simulink model "model"  (Simulink 7.5)
settings: Solver=ode23t  StartTime=0.0  StopTime=1  RelTol=1e-3
InitFcn:
  | sfunction_build
values from neighbouring files (symbols this model uses):
  D = 0.0001    [parameters.m]
  fx = 76.4e-3    (= 0.0764)    [parameters.m]
  J = 0.0001    [parameters.m]
  Lm = 0.0125    [parameters.m]
  P = 8    [parameters.m]
  Rs = 6.4    [parameters.m]
settings Model: Creator=mfilippa  LastModifiedBy=User
settings DebuggingCC: AlgebraicLoopMsg=error

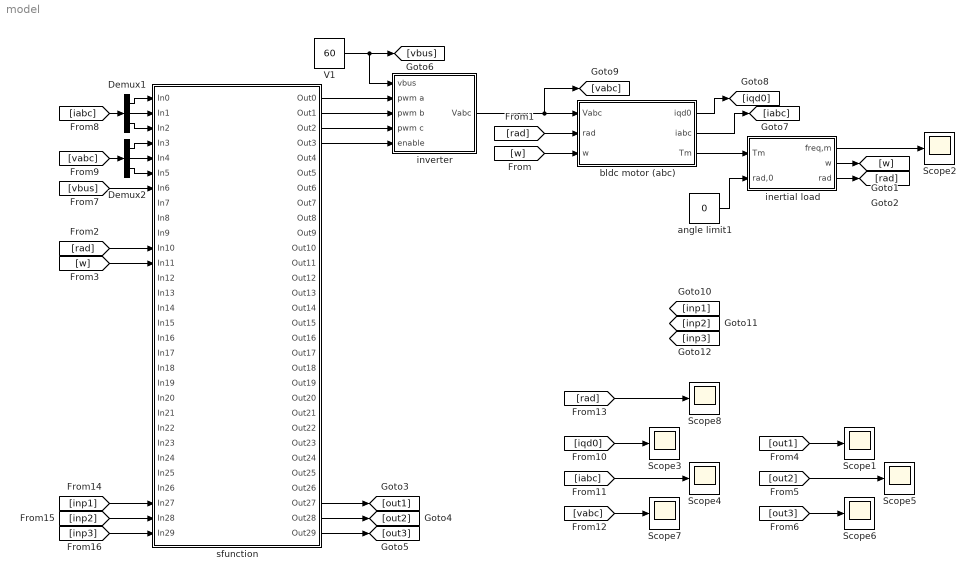
== system model ==
  Demux1 : Demux  Outputs=3
  Demux2 : Demux  Outputs=3
  Scope{1..8} (8 alike) : Scope
      Scope1 settings: YMin=8090  YMax=8230
      Scope3 settings: TimeRange=0.1722129783693844  YMin=-0.0402777777777777  YMax=0.06064814814814822  SaveName=ScopeData2
      Scope4 settings: SaveName=ScopeData3
      Scope5 settings: TimeRange=1.390547243523832e-005  YMin=7709.094650205756  YMax=7968.73799725651  SaveName=ScopeData4
      Scope6 settings: SaveName=ScopeData5
      Scope7 settings: SaveName=ScopeData6
      Scope8 settings: SaveName=ScopeData7
  V1 : Constant  Value=60
  angle limit1 : Constant  Value=0
  bldc motor (abc) : Subsystem
  inertial load : Subsystem
  inverter : Subsystem
  sfunction : Subsystem
  wires:
  V1/1 -> inverter/1(vbus), [vbus]
  sfunction/1(Out0) -> inverter/2(pwm a)
  sfunction/2(Out1) -> inverter/3(pwm b)
  sfunction/3(Out2) -> inverter/4(pwm c)
  sfunction/4(Out3) -> inverter/5(enable)
  [out1] -> Scope1/1
  inverter/1(Vabc) -> bldc motor (abc)/1(Vabc), [vabc]
  bldc motor (abc)/3(Tm) -> inertial load/1(Tm)
  [w] -> bldc motor (abc)/3(w)
  [rad] -> bldc motor (abc)/2(rad)
  inertial load/2(w) -> [w]
  inertial load/3(rad) -> [rad]
  [rad] -> sfunction/11(In10)
  [w] -> sfunction/12(In11)
  sfunction/30(Out29) -> [out3]
  sfunction/29(Out28) -> [out2]
  sfunction/28(Out27) -> [out1]
  [out2] -> Scope5/1
  [out3] -> Scope6/1
  [vbus] -> sfunction/7(In6)
  Demux1/1 -> sfunction/1(In0)
  Demux1/2 -> sfunction/2(In1)
  Demux1/3 -> sfunction/3(In2)
  [iabc] -> Demux1/1
  bldc motor (abc)/1(iqd0) -> [iqd0]
  bldc motor (abc)/2(iabc) -> [iabc]
  inertial load/1(freq,m) -> Scope2/1
  Demux2/1 -> sfunction/4(In3)
  Demux2/2 -> sfunction/5(In4)
  Demux2/3 -> sfunction/6(In5)
  [vabc] -> Demux2/1
  [iabc] -> Scope4/1
  [vabc] -> Scope7/1
  [iqd0] -> Scope3/1
  [inp1] -> sfunction/28(In27)
  [inp2] -> sfunction/29(In28)
  [inp3] -> sfunction/30(In29)
  [rad] -> Scope8/1
  angle limit1/1 -> inertial load/2(rad,0)

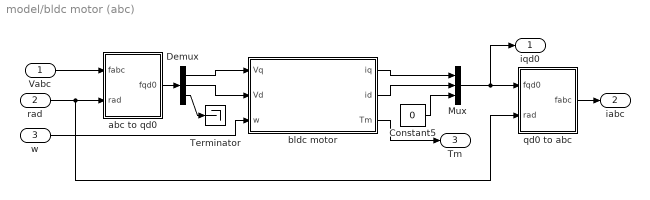
== system model/bldc motor (abc) ==
  Vabc : Inport  OutDataType=fixdt(1, 16)  OutScaling=2^0
  rad : Inport  Port=2  OutDataType=fixdt(1, 16)  OutScaling=2^0
  w : Inport  Port=3  OutDataType=fixdt(1, 16)  OutScaling=2^0
  Constant5 : Constant  Value=0  OutDataType=fixdt(1, 16)  OutScaling=2^0
  Demux : Demux  Outputs=3
  Mux : Mux  Inputs=3
  Terminator : Terminator
  abc to qd0 : Subsystem
  bldc motor : Subsystem
  qd0 to abc : Subsystem
  iqd0 : Outport  OutDataType=fixdt(1, 16)  OutScaling=2^0
  iabc : Outport  Port=2  OutDataType=fixdt(1, 16)  OutScaling=2^0
  Tm : Outport  Port=3  OutDataType=fixdt(1, 16)  OutScaling=2^0
  wires:
  abc to qd0/1(fqd0) -> Demux/1
  Demux/1 -> bldc motor/1(Vq)
  Demux/2 -> bldc motor/2(Vd)
  bldc motor/1(iq) -> Mux/1
  bldc motor/2(id) -> Mux/2
  Mux/1 -> qd0 to abc/1(fqd0), iqd0/1
  Constant5/1 -> Mux/3
  Vabc/1 -> abc to qd0/1(fabc)
  rad/1 -> abc to qd0/2(rad), qd0 to abc/2(rad)
  w/1 -> bldc motor/3(w)
  qd0 to abc/1(fabc) -> iabc/1
  bldc motor/3(Tm) -> Tm/1
  Demux/3 -> Terminator/1

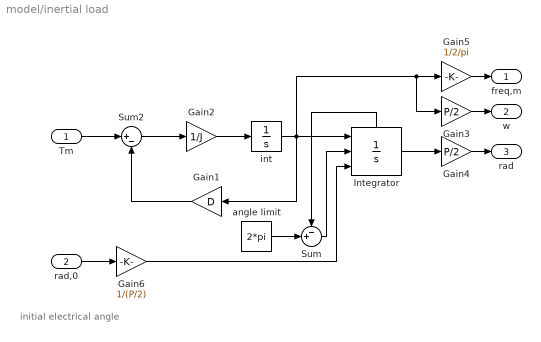
== system model/inertial load ==
  note: initial
      | electrical
      | angle
  Tm : Inport
  rad,0 : Inport  Port=2
  Gain1 : Gain  Gain=D  ParameterDataType=fixdt(1, 16)  ParameterScaling=2^0  OutDataType=fixdt(1, 16)  OutScaling=2^0
  Gain2 : Gain  Gain=1/J  ParameterDataType=fixdt(1, 16)  ParameterScaling=2^0  OutDataType=fixdt(1, 16)  OutScaling=2^0
  Gain3 : Gain  Gain=P/2  ParameterDataType=fixdt(1, 16)  ParameterScaling=2^0  OutDataType=fixdt(1, 16)  OutScaling=2^0
  Gain4 : Gain  Gain=P/2  ParameterDataType=fixdt(1, 16)  ParameterScaling=2^0  OutDataType=fixdt(1, 16)  OutScaling=2^0
  Gain5 : Gain  Gain=1/2/pi  ParameterDataType=fixdt(1, 16)  ParameterScaling=2^0  OutDataType=fixdt(1, 16)  OutScaling=2^0
  Gain6 : Gain  Gain=1/(P/2)  ParameterDataType=fixdt(1, 16)  ParameterScaling=2^0  OutDataType=fixdt(1, 16)  OutScaling=2^0
  Integrator : Integrator  ExternalReset=falling  InitialConditionSource=external  ShowStatePort=on
  Sum : Sum  Inputs=-+|
  Sum2 : Sum  Inputs=|+-  OutDataType=fixdt(1, 16)  OutScaling=2^0
  angle limit : Constant  Value=2*pi
  int : Integrator
  freq,m : Outport  OutDataType=fixdt(1, 16)  OutScaling=2^0
  w : Outport  Port=2  OutDataType=fixdt(1, 16)  OutScaling=2^0
  rad : Outport  Port=3  OutDataType=fixdt(1, 16)  OutScaling=2^0
  wires:
  Gain1/1 -> Sum2/2
  Integrator/1 -> Gain4/1
  Integrator/State -> Sum/1
  angle limit/1 -> Sum/2
  Sum/1 -> Integrator/2
  int/1 -> Gain1/1, Integrator/1, Gain3/1, Gain5/1
  Gain2/1 -> int/1
  Sum2/1 -> Gain2/1
  Tm/1 -> Sum2/1
  Gain3/1 -> w/1
  Gain4/1 -> rad/1
  Gain5/1 -> freq,m/1
  Gain6/1 -> Integrator/3
  rad,0/1 -> Gain6/1

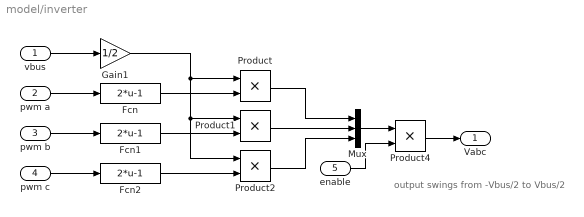
== system model/inverter ==
  note: output swings from
      | -Vbus/2 to Vbus/2
  vbus : Inport  OutDataType=fixdt(1, 16)  OutScaling=2^0
  pwm a : Inport  Port=2  OutDataType=fixdt(1, 16)  OutScaling=2^0
  pwm b : Inport  Port=3  OutDataType=fixdt(1, 16)  OutScaling=2^0
  pwm c : Inport  Port=4  OutDataType=fixdt(1, 16)  OutScaling=2^0
  enable : Inport  Port=5  OutDataType=fixdt(1, 16)  OutScaling=2^0
  Fcn : Fcn  Expr=2*u-1
  Fcn1 : Fcn  Expr=2*u-1
  Fcn2 : Fcn  Expr=2*u-1
  Gain1 : Gain  Gain=1/2  ParameterDataType=fixdt(1, 16)  ParameterScaling=2^0  OutDataType=fixdt(1, 16)  OutScaling=2^0
  Mux : Mux  Inputs=3
  Product{,1..2,4} (4 alike) : Product  OutDataType=fixdt(1, 16)  OutScaling=2^0  RndMeth=Zero
  Vabc : Outport  OutDataType=fixdt(1, 16)  OutScaling=2^0
  wires:
  vbus/1 -> Gain1/1
  Product/1 -> Mux/1
  Product1/1 -> Mux/2
  Product2/1 -> Mux/3
  Fcn/1 -> Product/2
  Fcn1/1 -> Product1/2
  Fcn2/1 -> Product2/2
  Gain1/1 -> Product/1, Product1/1, Product2/1
  pwm a/1 -> Fcn/1
  pwm b/1 -> Fcn1/1
  pwm c/1 -> Fcn2/1
  Mux/1 -> Product4/1
  Product4/1 -> Vabc/1
  enable/1 -> Product4/2

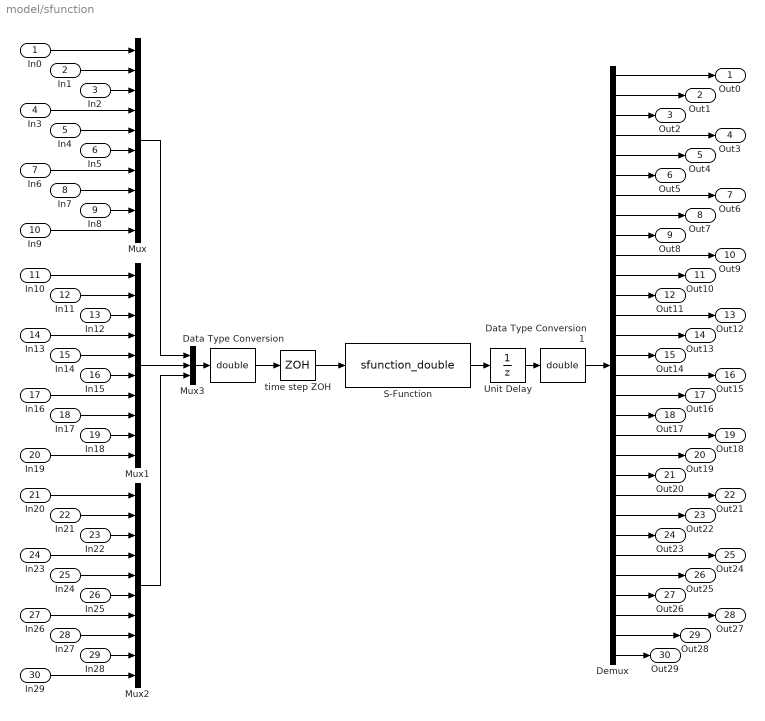
== system model/sfunction ==
  In0 : Inport
  In1 : Inport  Port=2
  In2 : Inport  Port=3
  In3 : Inport  Port=4
  In4 : Inport  Port=5
  In5 : Inport  Port=6
  In6 : Inport  Port=7
  In7 : Inport  Port=8
  In8 : Inport  Port=9
  In9 : Inport  Port=10
  In10 : Inport  Port=11
  In11 : Inport  Port=12
  In12 : Inport  Port=13
  In13 : Inport  Port=14
  In14 : Inport  Port=15
  In15 : Inport  Port=16
  In16 : Inport  Port=17
  In17 : Inport  Port=18
  In18 : Inport  Port=19
  In19 : Inport  Port=20
  In20 : Inport  Port=21
  In21 : Inport  Port=22
  In22 : Inport  Port=23
  In23 : Inport  Port=24
  In24 : Inport  Port=25
  In25 : Inport  Port=26
  In26 : Inport  Port=27
  In27 : Inport  Port=28
  In28 : Inport  Port=29
  In29 : Inport  Port=30
  Data Type Conversion : DataTypeConversion  OutDataTypeMode=double  OutDataTypeStr=double
  Data Type Conversion1 : DataTypeConversion  OutDataTypeMode=double  OutDataTypeStr=double
  Demux : Demux  Outputs=30
  Mux : Mux  Inputs=10
  Mux1 : Mux  Inputs=10
  Mux2 : Mux  Inputs=10
  Mux3 : Mux  Inputs=3
  S-Function : S-Function  FunctionName=sfunction_double  EnableBusSupport=off
  Unit Delay : UnitDelay  SampleTime=-1
  time step ZOH : ZeroOrderHold  SampleTime=1/8000
  Out0 : Outport
  Out1 : Outport  Port=2
  Out2 : Outport  Port=3
  Out3 : Outport  Port=4
  Out4 : Outport  Port=5
  Out5 : Outport  Port=6
  Out6 : Outport  Port=7
  Out7 : Outport  Port=8
  Out8 : Outport  Port=9
  Out9 : Outport  Port=10
  Out10 : Outport  Port=11
  Out11 : Outport  Port=12
  Out12 : Outport  Port=13
  Out13 : Outport  Port=14
  Out14 : Outport  Port=15
  Out15 : Outport  Port=16
  Out16 : Outport  Port=17
  Out17 : Outport  Port=18
  Out18 : Outport  Port=19
  Out19 : Outport  Port=20
  Out20 : Outport  Port=21
  Out21 : Outport  Port=22
  Out22 : Outport  Port=23
  Out23 : Outport  Port=24
  Out24 : Outport  Port=25
  Out25 : Outport  Port=26
  Out26 : Outport  Port=27
  Out27 : Outport  Port=28
  Out28 : Outport  Port=29
  Out29 : Outport  Port=30
  wires:
  Data Type Conversion/1 -> time step ZOH/1
  In9/1 -> Mux/10
  In8/1 -> Mux/9
  In7/1 -> Mux/8
  In6/1 -> Mux/7
  In5/1 -> Mux/6
  In4/1 -> Mux/5
  In3/1 -> Mux/4
  In2/1 -> Mux/3
  In1/1 -> Mux/2
  In0/1 -> Mux/1
  time step ZOH/1 -> S-Function/1
  In19/1 -> Mux1/10
  In18/1 -> Mux1/9
  In17/1 -> Mux1/8
  In16/1 -> Mux1/7
  In15/1 -> Mux1/6
  In14/1 -> Mux1/5
  In13/1 -> Mux1/4
  In12/1 -> Mux1/3
  In11/1 -> Mux1/2
  In10/1 -> Mux1/1
  In29/1 -> Mux2/10
  In28/1 -> Mux2/9
  In27/1 -> Mux2/8
  In26/1 -> Mux2/7
  In25/1 -> Mux2/6
  In24/1 -> Mux2/5
  In23/1 -> Mux2/4
  In22/1 -> Mux2/3
  In21/1 -> Mux2/2
  In20/1 -> Mux2/1
  Mux3/1 -> Data Type Conversion/1
  Mux/1 -> Mux3/1
  Mux2/1 -> Mux3/3
  Mux1/1 -> Mux3/2
  Demux/1 -> Out0/1
  Demux/2 -> Out1/1
  Demux/3 -> Out2/1
  Demux/4 -> Out3/1
  Demux/5 -> Out4/1
  Demux/6 -> Out5/1
  Demux/7 -> Out6/1
  Demux/8 -> Out7/1
  Demux/9 -> Out8/1
  Demux/10 -> Out9/1
  Demux/11 -> Out10/1
  Demux/12 -> Out11/1
  Demux/13 -> Out12/1
  Demux/14 -> Out13/1
  Demux/15 -> Out14/1
  Demux/16 -> Out15/1
  Demux/17 -> Out16/1
  Demux/18 -> Out17/1
  Demux/19 -> Out18/1
  Demux/20 -> Out19/1
  Demux/21 -> Out20/1
  Demux/22 -> Out21/1
  Demux/23 -> Out22/1
  Demux/24 -> Out23/1
  Demux/25 -> Out24/1
  Demux/26 -> Out25/1
  Demux/27 -> Out26/1
  Demux/28 -> Out27/1
  Demux/29 -> Out28/1
  Demux/30 -> Out29/1
  S-Function/1 -> Unit Delay/1
  Data Type Conversion1/1 -> Demux/1
  Unit Delay/1 -> Data Type Conversion1/1

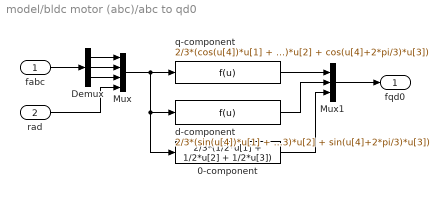
== system model/bldc motor (abc)/abc to qd0 ==
  fabc : Inport
  rad : Inport  Port=2
  0-component : Fcn  Expr=2/3*(1/2*u[1] + 1/2*u[2] + 1/2*u[3])
  Demux : Demux  Outputs=3
  Mux : Mux
  Mux1 : Mux  Inputs=3
  d-component : Fcn  Expr=2/3*(sin(u[4])*u[1] + sin(u[4]-2*pi/3)*u[2] + sin(u[4]+2*pi/3)*u[3])
  q-component : Fcn  Expr=2/3*(cos(u[4])*u[1] + cos(u[4]-2*pi/3)*u[2] + cos(u[4]+2*pi/3)*u[3])
  fqd0 : Outport
  wires:
  Mux/1 -> 0-component/1, d-component/1, q-component/1
  rad/1 -> Mux/4
  fabc/1 -> Demux/1
  Demux/1 -> Mux/1
  Demux/2 -> Mux/2
  Demux/3 -> Mux/3
  q-component/1 -> Mux1/1
  d-component/1 -> Mux1/2
  0-component/1 -> Mux1/3
  Mux1/1 -> fqd0/1

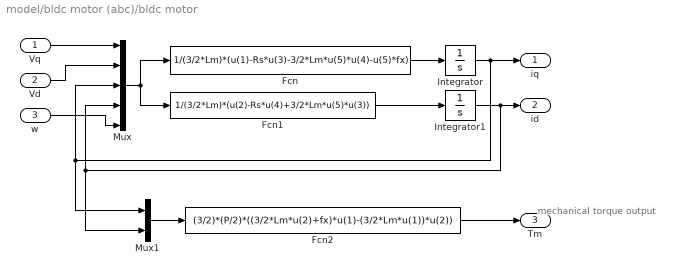
== system model/bldc motor (abc)/bldc motor ==
  note: mechanical
      | torque output
  Vq : Inport
  Vd : Inport  Port=2
  w : Inport  Port=3
  Fcn : Fcn  Expr=1/(3/2*Lm)*(u(1)-Rs*u(3)-3/2*Lm*u(5)*u(4)-u(5)*fx)
  Fcn1 : Fcn  Expr=1/(3/2*Lm)*(u(2)-Rs*u(4)+3/2*Lm*u(5)*u(3))
  Fcn2 : Fcn  Expr=(3/2)*(P/2)*((3/2*Lm*u(2)+fx)*u(1)-(3/2*Lm*u(1))*u(2))
  Integrator : Integrator
  Integrator1 : Integrator
  Mux : Mux  Inputs=5
  Mux1 : Mux  Inputs=2
  iq : Outport  OutDataType=fixdt(1, 16)  OutScaling=2^0
  id : Outport  Port=2  OutDataType=fixdt(1, 16)  OutScaling=2^0
  Tm : Outport  Port=3  OutDataType=fixdt(1, 16)  OutScaling=2^0
  wires:
  Fcn1/1 -> Integrator1/1
  Fcn/1 -> Integrator/1
  Integrator/1 -> iq/1, Mux/3, Mux1/1
  Integrator1/1 -> id/1, Mux1/2, Mux/4
  Mux1/1 -> Fcn2/1
  Fcn2/1 -> Tm/1
  Vq/1 -> Mux/1
  Mux/1 -> Fcn/1, Fcn1/1
  Vd/1 -> Mux/2
  w/1 -> Mux/5

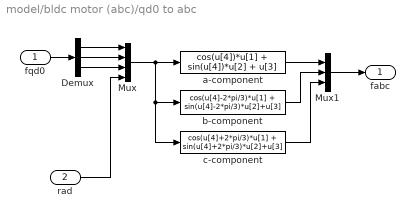
== system model/bldc motor (abc)/qd0 to abc ==
  fqd0 : Inport
  rad : Inport  Port=2
  Demux : Demux  Outputs=3
  Mux : Mux
  Mux1 : Mux  Inputs=3
  a-component : Fcn  Expr=cos(u[4])*u[1] + sin(u[4])*u[2] + u[3]
  b-component : Fcn  Expr=cos(u[4]-2*pi/3)*u[1] + sin(u[4]-2*pi/3)*u[2]+u[3]
  c-component : Fcn  Expr=cos(u[4]+2*pi/3)*u[1] + sin(u[4]+2*pi/3)*u[2]+u[3]
  fabc : Outport
  wires:
  rad/1 -> Mux/4
  Mux/1 -> a-component/1, b-component/1, c-component/1
  fqd0/1 -> Demux/1
  Demux/1 -> Mux/1
  Demux/2 -> Mux/2
  Demux/3 -> Mux/3
  a-component/1 -> Mux1/1
  b-component/1 -> Mux1/2
  Mux1/1 -> fabc/1
  c-component/1 -> Mux1/3
